simulink model "body_frame_iopid"  (R2017a)
settings: Solver=FixedStepAuto  StartTime=0.0  StopTime=100  FixedStep=0.01  RelTol=1e-3
undefined symbols (not defined in the file): CoordinateFrame, TypeMask, Velocity
libraries: robotlib x3, simulink x1
settings Model: Creator=bshang2  LastModifiedBy=bshang2

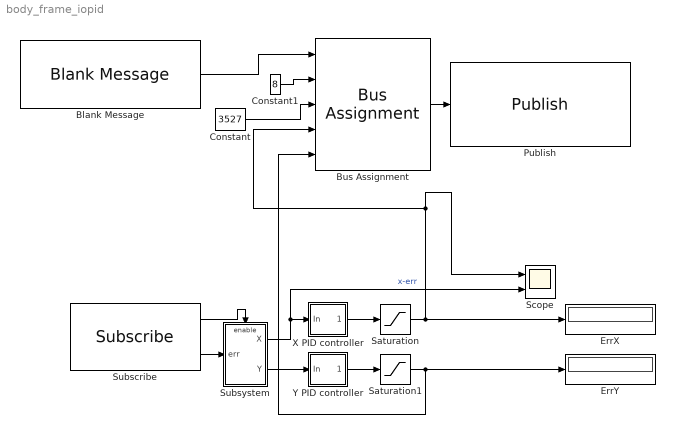
== system body_frame_iopid ==
  Blank Message : robotlib/Blank Message  SourceLibraryInfo=This block requires Robotics System Toolbox  messageType=mavros_msgs/PositionTarget  SampleTime=inf
      settings: SourceProductBaseCode=RO
  Bus Assignment : BusAssignment  AssignedSignals=CoordinateFrame,TypeMask,Velocity.X,Velocity.Y
  Constant : Constant  Value=3527  OutDataTypeStr=uint16
  Constant1 : Constant  Value=8  OutDataTypeStr=uint8
  ErrX : Display
  ErrY : Display
  Publish : robotlib/Publish  SourceLibraryInfo=This block requires Robotics System Toolbox  topicSource=Select from ROS network  topic=/mavros/setpoint_raw/local  messageType=mavros_msgs/PositionTarget  messageQueueLength=1
      settings: SourceProductBaseCode=RO
  Saturation : Saturate  UpperLimit=0.3  LowerLimit=-0.3
  Saturation1 : Saturate  UpperLimit=0.3  LowerLimit=-0.3
  Scope : Scope  NumInputPorts=2
  Subscribe : robotlib/Subscribe  SourceLibraryInfo=This block requires Robotics System Toolbox  topicSource=Select from ROS network  topic=/matlab/err  messageType=geometry_msgs/Pose2D  sampleTime=-1  messageQueueLength=1
      settings: SourceProductBaseCode=RO
  Subsystem : Subsystem
  X PID controller : Subsystem
  Y PID controller : Subsystem
  wires:
  Blank Message/1 -> Bus Assignment/1
  Saturation/1 -> ErrX/1, Bus Assignment/4, Scope/1
  Bus Assignment/1 -> Publish/1
  Subscribe/2 -> Subsystem/1(err)
  Subsystem/1(X) -> Scope/2, X PID controller/1(In)  "x-err"
  Subsystem/2(Y) -> Y PID controller/1(In)
  Subscribe/1 -> Subsystem/Enable
  Y PID controller/1(Out) -> Saturation1/1
  Saturation1/1 -> Bus Assignment/5, ErrY/1
  Constant/1 -> Bus Assignment/3
  Constant1/1 -> Bus Assignment/2
  X PID controller/1(Out) -> Saturation/1

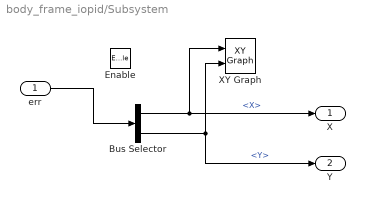
== system body_frame_iopid/Subsystem ==
  err : Inport
  Enable : EnablePort
  Bus Selector : BusSelector  OutputSignals=X,Y
  XY Graph : simulink/Sinks/XY Graph  xmin=-100  xmax=100  ymin=-100  ymax=100  st=-1
  X : Outport
  Y : Outport  Port=2
  wires:
  err/1 -> Bus Selector/1
  Bus Selector/1 -> X/1, XY Graph/1  "<X>"
  Bus Selector/2 -> Y/1, XY Graph/2  "<Y>"

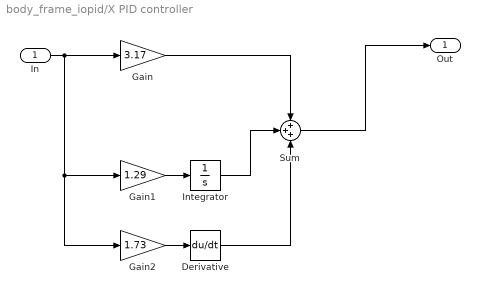
== system body_frame_iopid/X PID controller ==
  In : Inport
  Derivative : Derivative
  Gain : Gain  Gain=3.17
  Gain1 : Gain  Gain=1.29
  Gain2 : Gain  Gain=1.73
  Integrator : Integrator
  Sum : Sum  Inputs=+++
  Out : Outport
  wires:
  Sum/1 -> Out/1
  In/1 -> Gain1/1, Gain2/1, Gain/1
  Gain1/1 -> Integrator/1
  Gain2/1 -> Derivative/1
  Gain/1 -> Sum/1
  Integrator/1 -> Sum/2
  Derivative/1 -> Sum/3

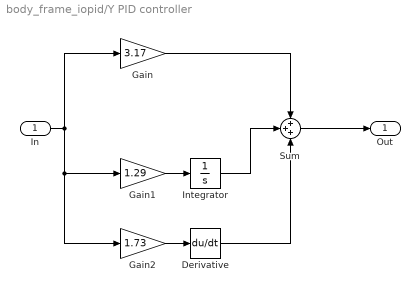
== system body_frame_iopid/Y PID controller ==
  In : Inport
  Derivative : Derivative
  Gain : Gain  Gain=3.17
  Gain1 : Gain  Gain=1.29
  Gain2 : Gain  Gain=1.73
  Integrator : Integrator
  Sum : Sum  Inputs=+++
  Out : Outport
  wires:
  Sum/1 -> Out/1
  In/1 -> Gain/1, Gain1/1, Gain2/1
  Gain1/1 -> Integrator/1
  Gain2/1 -> Derivative/1
  Gain/1 -> Sum/1
  Integrator/1 -> Sum/2
  Derivative/1 -> Sum/3
